simulink model "untitled2"  (R2024b)
settings: Solver=VariableStepAuto  StartTime=0.0  StopTime=10.0  MaxStep=5  RelTol=1e-3
values from neighbouring files (symbols this model uses):
  Cvl = Cp * rop * Vl    (= 30000)    [MocGrzalkiPI.m]    (also in PrawyCz1.m; PrawyCz2.m; Spr2.m; Sprb.m)
  Cvp = Cp * rop * Vp    (= 150000)    [MocGrzalkiPI.m]    (also in PrawyCz1.m; PrawyCz2.m; Spr2.m; Sprb.m)
  czasskok = 500    [Lab5.m]    (also in MocGrzalkiPI.m; PrawyCz1.m = 0; PrawyCz2.m; Spr2.m = 1000)
  delta_Pg = 1.1    [MocGrzalkiPI.m]    (also in PrawyCz1.m; PrawyCz2.m; Spr2.m = 1000; Sprb.m)
  deltaTzew = 5    [MocGrzalkiPI.m]    (also in PrawyCz1.m = 0; PrawyCz2.m = 0; Spr2.m = 0; Sprb.m = 0)
  dSP = 0    [MocGrzalkiPI.m]    (also in gpt02.m; labPI.m = 1)
  Kp = 0.9 * T / (k * Tzero)    (= 4885.71428571)    [MocGrzalkiPI.m]    (also in gpt02.m; labPI.m)
  Ksl = a * Ksp    (= 173.913043478)    [MocGrzalkiPI.m]    (also in PrawyCz1.m; PrawyCz2.m; Spr2.m; Sprb.m)
  Ksp = Pgn / (a * (Tl_nominal - TzewN) + (Tp_nominal - TzewN))    (= 86.9565217391)    [MocGrzalkiPI.m]    (also in PrawyCz1.m; PrawyCz2.m; Spr2.m; Sprb.m)
  Ksw = Ksp * (Tp_nominal - TzewN) / (Tl_nominal - Tp_nominal)    (= 608.695652174)    [MocGrzalkiPI.m]    (also in PrawyCz1.m; PrawyCz2.m; Spr2.m; Sprb.m)
  Pg0 = Pgn    (= 10000)    [MocGrzalkiPI.m]    (also in PrawyCz1.m; PrawyCz2.m; Spr2.m; Sprb.m)
  SP0 = Tp_eq    [MocGrzalkiPI.m]    (also in labPI.m)
  Ti = 3.33 * Tzero    (= 133.2)    [MocGrzalkiPI.m]    (also in gpt02.m; labPI.m)
  Tl_eq = Temps(1)    [MocGrzalkiPI.m]    (also in PrawyCz1.m; PrawyCz2.m; Spr2.m; dziala.m)
  Tp_eq = Temps(2)    [MocGrzalkiPI.m]    (also in PrawyCz1.m; PrawyCz2.m; Spr2.m; dziala.m)
  Tzew0 = TzewN    (= -20)    [MocGrzalkiPI.m]    (also in PrawyCz1.m; PrawyCz2.m; Spr2.m; dziala.m = tab_Tzew0(i))
settings Model: Creator=pawli  LastModifiedBy=pawli

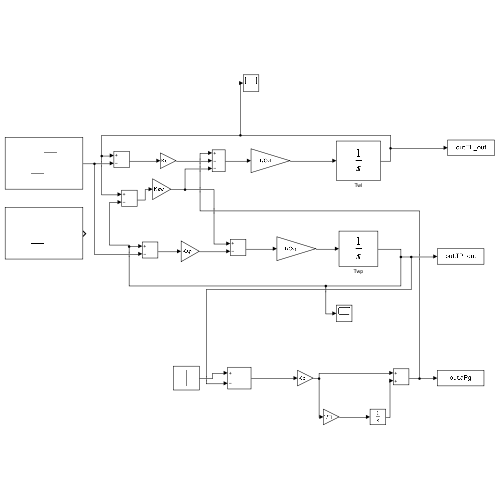
[thumbnail: Simulink's stored preview of the top-level diagram]
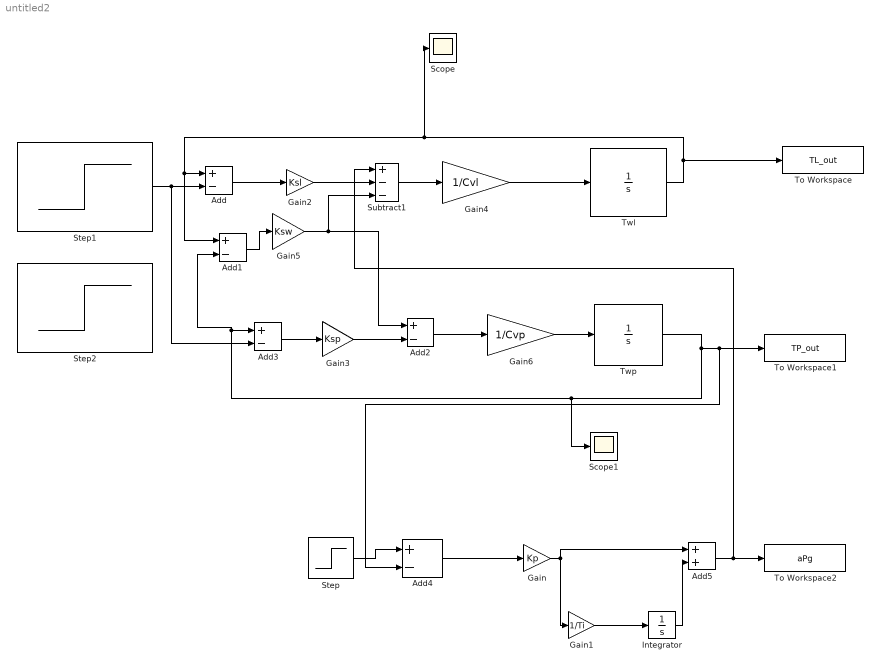
== system untitled2 ==
  Add{,1..4} (5 alike) : Sum  Inputs=+-
  Add5 : Sum
  Gain : Gain  Gain=Kp
  Gain1 : Gain  Gain=1/Ti
  Gain2 : Gain  Gain=Ksl
  Gain3 : Gain  Gain=Ksp
  Gain4 : Gain  Gain=1/Cvl
  Gain5 : Gain  Gain=Ksw
  Gain6 : Gain  Gain=1/Cvp
  Integrator : Integrator  InitialCondition=Pg0
  Scope : Scope
  Scope1 : Scope
  Step : Step  Time=czasskok  Before=SP0  After=SP0+dSP  SampleTime=0
  Step1 : Step  Time=czasskok  Before=Tzew0  After=Tzew0+deltaTzew  SampleTime=0
  Step2 : Step  Time=czasskok  Before=Pg0  After=Pg0 * delta_Pg  SampleTime=0
  Subtract1 : Sum  Inputs=+--
  To Workspace : ToWorkspace  VariableName=TL_out  SampleTime=-1
  To Workspace1 : ToWorkspace  VariableName=TP_out  SampleTime=-1
  To Workspace2 : ToWorkspace  VariableName=aPg  SampleTime=-1
  Twl : Integrator  InitialCondition=Tl_eq
  Twp : Integrator  InitialCondition=Tp_eq
  wires:
  Step/1 -> Add4/1
  Add4/1 -> Gain/1
  Gain/1 -> Add5/1, Gain1/1
  Gain1/1 -> Integrator/1
  Integrator/1 -> Add5/2
  Gain5/1 -> Add2/1, Subtract1/3
  Add3/1 -> Gain3/1
  Add/1 -> Gain2/1
  Twl/1 -> To Workspace/1, Scope/1, Add1/1, Add/1
  Step1/1 -> Add3/2, Add/2
  Add2/1 -> Gain6/1
  Twp/1 -> Scope1/1, Add3/1, Add1/2, Add4/2, To Workspace1/1
  Gain2/1 -> Subtract1/2
  Subtract1/1 -> Gain4/1
  Gain6/1 -> Twp/1
  Gain3/1 -> Add2/2
  Gain4/1 -> Twl/1
  Add1/1 -> Gain5/1
  Add5/1 -> Subtract1/1, To Workspace2/1
